simulink library "tqd"  (R2021b)
settings: Solver=VariableStepAuto  StartTime=0.0  StopTime=10.0  RelTol=1e-3
undefined symbols (not defined in the file): ATQD_AfterTqMinGain_X_Deg, ATQD_APSCreepBaseTqD_X_kph, ATQD_APSCreepBaseTqD_Y_Deg, ATQD_APSCreepBaseTqR_X_kph, ATQD_APSCreepBaseTqR_Y_Deg, ATQD_APSCreepIterm_X_kph, ATQD_APSCreepIterm_Y_kph, ATQD_APSCreepPterm_X_kph, ATQD_APSCreepPterm_Y_kph, ATQD_APSDecReq_X_kph, ATQD_APSDecReq_Y_mps2, ATQD_APSDecReqCMD_X_kph, ATQD_APSDecReqTs_X_pct, ATQD_APSDecTimeGain_X_Deg, ATQD_APSDecTimeGain_Y_s, ATQD_APSReqLowSpd_X_Deg, ATQD_AutoHoldReleaseBPS_X_Deg, ATQD_AWDLoadTrqnsGain_X_kg, ATQD_AWDLoadTrqnsGain_Y_pct, ATQD_BOSEnBPSPosn_X_kph, ATQD_BOSMap_X_rpm, ATQD_BOSMap_Y_pct, ATQD_CreepBaseTqD_X_kph, ATQD_CreepBaseTqD_Y_Deg, ATQD_CreepBaseTqR_X_kph, ATQD_CreepBaseTqR_Y_Deg, ATQD_CreepBPSDisPosn_X_Deg, ATQD_CreepBPSDisPosnR_X_Deg, ATQD_CreepBPSEnPosn_X_Deg, ATQD_CreepBPSEnPosnR_X_Deg, ATQD_CreepDeltaTq_X_kph, ATQD_CreepIterm_X_kph, ATQD_CreepIterm_Y_kph, ATQD_CreepItermMaxLimit_X_pct, ATQD_CreepPreloadTime_X_kph, ATQD_CreepPreloadTq_X_kph, ATQD_CreepPreloadTq_Y_s, ATQD_CreepProtTq_X_Deg, ATQD_CreepPterm_X_kph, ATQD_CreepPterm_Y_kph, ATQD_CreepRrTqSpRat_X_rpm, ATQD_CreepRrTqSpRat_Y_Nm, ATQD_CreepTargetSpdD_X_pct, ATQD_CreepTargetSpdR_X_pct, ATQD_ECOTqMapD_X_rpm, ATQD_ECOTqMapD_Y_pct, ATQD_EMTqMapD_X_rpm, ATQD_EMTqMapD_Y_pct, ATQD_EOPDTqMapDCon_X_rpm, ATQD_EOPDTqMapDCon_Y_Deg, ATQD_EscapeModePedTq_X_pct, ATQD_EscapeModePedTq_Y_rpm, ATQD_EscapeModePedTqFr_X_pct, ATQD_EscapeModePedTqFr_Y_rpm, ATQD_EstInitVehWeight_X_c, ATQD_FAfterTqCMDGain_X_rpm, ATQD_FAfterTqCMDGain_Y_pct, ATQD_FrLossMAPLowV_X_rpm, ATQD_FrLossMAPLowV_Y_Nm, ATQD_FrMotActReduce_X_rpm ... (+772)
libraries: simulink x211, hcu_lib x179, tqr x3
(part 7 of 28)

== system tqd/TQD/TorqueDemand/Signal_convert/SWC2_Subsystem ==
  note: Speed Setting Mode
  note: Speed Control Mode
  note: Fail safe switch
  VINP_SWC2LScrollUpSta_flg : Inport
  VINP_SWC2LScrollDownSta_flg : Inport  Port=2
  VINP_SWC2LScrollPressSta_flg : Inport  Port=3
  VINP_SWC2LADASSta_flg : Inport  Port=4
  VTQD_GearActualPosn_enum : Inport  Port=5
  VVMC_ADASActive_flg : Inport  Port=6
  VVMC_LVDAACCStaInfor_flg : Inport  Port=7
  VVMC_MSAActive_flg : Inport  Port=8
  VINP_ADASACCSta_enum : Inport  Port=9
  VVMC_MeterIndSpeed_raw32 : Inport  Port=10
  VINP_ADASSLIFSpdLim_enum : Inport  Port=11
  task_time_s : Inport  Port=12
  VINP_IVIISAOffsetSpd_enum : Inport  Port=13
  VPMM_PowerSta_enum : Inport  Port=14
  VTQD_ShiftGearPosn_enum : Inport  Port=15
  VVMC_MSACtrlSta_enum : Inport  Port=16
  VINP_VehSpeed_kph : Inport  Port=17
  VINP_Distanceunit_flg : Inport  Port=18
  VINP_IVIACCAdaptiveSta_flg : Inport  Port=19
  VVMC_CCCtrlSta_enum : Inport  Port=20
  VVMC_ACCObjDist_m : Inport  Port=21
  VINP_SmartEcoModeSW_flg : Inport  Port=22
  VVMC_SetACCDisableAPS_flg : Inport  Port=23
  VINP_SWCRegenUp_flg : Inport  Port=24
  VINP_SWCRegenDown_flg : Inport  Port=25
  VINP_SWC2RScrollUpSta_flg : Inport  Port=26
  VINP_SWC2RScrollDownSta_flg : Inport  Port=27
  VINP_SWC2LDriveModeSta_flg : Inport  Port=28
  VINP_SWC2RScrollPressSta_flg : Inport  Port=29
  VINP_SWC2RRightSta_flg : Inport  Port=30
  VINP_SWC2RLeftSta_flg : Inport  Port=31
  VTQD_LowIdleAccPedal_flg : Inport  Port=32
  Enable : EnablePort
  AND1 : Logic  AllPortsSameDT=off  OutDataTypeStr=boolean
  AND{8,10,12..13,17..18} (6 alike) : Logic  Inputs=3  AllPortsSameDT=off  OutDataTypeStr=boolean
  AND11 : Logic  Inputs=4  AllPortsSameDT=off  OutDataTypeStr=boolean
  AND14 : Logic  Operator=OR  AllPortsSameDT=off  OutDataTypeStr=boolean
  AND16 : Logic  Operator=OR  AllPortsSameDT=off  OutDataTypeStr=boolean
  AND6 : Logic  AllPortsSameDT=off  OutDataTypeStr=boolean
  Add1 : Sum
  Big Mike Combo : Subsystem  AncestorBlock=tqd0/TQD/TorqueDemand/Signal_convert/Big Mike Combo
  Constant1 : Constant  Value=ENUM_ADASACCSTA_OVERRIDE
  Constant{89,92,94..95,110..113} (8 alike) : Constant  Value=FALSE
  Constant116 : Constant  Value=ENUM_GEARACTUALPOSN_D
  Constant117 : Constant  Value=ENUM_SWCBOTTONPRESS_LONGPRESS
  Constant118 : Constant  Value=ENUM_GEARACTUALPOSN_D
  Constant119 : Constant  Value=ENUM_SPDCTRLMODE_MSA
  Constant120 : Constant  Value=ENUM_SWCBOTTONPRESS_SHORTPRESS
  Constant121 : Constant  Value=KTQD_OvrSpdSetDownOffSet_kph
  Constant122 : Constant  Value=ENUM_SWCBOTTONPRESS_LONGPRESS
  Constant123 : Constant  Value=ENUM_SWCBOTTONPRESS_SHORTPRESS
  Constant124 : Constant  Value=ENUM_ADASACCSTA_ACTIVE
  Constant125 : Constant  Value=ENUM_ADASACCSTA_ACTIVE
  Constant126 : Constant  Value=0x0  OutDataTypeStr=uint8
  Constant127 : Constant  Value=ENUM_SPDCTRLMODE_MSA
  Constant128 : Constant  Value=ENUM_SPDCTRLMODE_ACC
  Constant129 : Constant  Value=ENUM_GEARACTUALPOSN_D
  Constant130 : Constant  Value=ENUM_SPDCTRLMODE_MSA
  Constant77 : Constant  Value=KTQD_SpdCtrlMode_enum_ovrdflg
  Constant78 : Constant  Value=KTQD_SpdCtrlMode_enum_ovrdval
  Constant82 : Constant  Value=KTQD_Veh2MetSpdLowBand_kph
  Constant84 : Constant  Value=KTQD_Veh2MetSpdHiBand_kph
  Constant90 : Constant  Value=ENUM_POWERSTA_READY
  Constant91 : Constant  Value=ENUM_SPDCTRLMODE_OFF
  Data Type Conversion4 : DataTypeConversion  OutDataTypeStr=single
  Delay{5..6,10..13} (6 alike) : Delay  DelayLength=1
  Detect Decrease2 : simulink/Logic and Bit Operations/Detect Decrease  vinit=0.0  OutDataTypeStr=boolean
  Detect Increase1 : simulink/Logic and Bit Operations/Detect Increase  vinit=0.0  OutDataTypeStr=boolean
  Detect Increase2 : simulink/Logic and Bit Operations/Detect Increase  vinit=0.0  OutDataTypeStr=boolean
  Equal{1,30,41..48,50,52} (12 alike) : RelationalOperator  Operator===  OutDataTypeStr=boolean  RndMeth=Simplest
  Equal{40,49,51,53} (4 alike) : RelationalOperator  Operator=~=  OutDataTypeStr=boolean  RndMeth=Simplest
  L_ScrollPress Behavior : Subsystem
  NOT{1..4} (4 alike) : Logic  Operator=NOT  AllPortsSameDT=off  OutDataTypeStr=boolean
  OR2 : Logic  Operator=OR  Inputs=4  AllPortsSameDT=off  OutDataTypeStr=boolean
  OR{3..8} (6 alike) : Logic  Operator=OR  AllPortsSameDT=off  OutDataTypeStr=boolean
  Relational Operator2 : RelationalOperator  OutDataTypeStr=boolean  RndMeth=Simplest
  Relational Operator3 : RelationalOperator  Operator=>  OutDataTypeStr=boolean  RndMeth=Simplest
  Relational Operator6 : RelationalOperator  Operator=<=  OutDataTypeStr=boolean  RndMeth=Simplest
  Road Speed Limit Convert : Subsystem
  SR_Latch4 : hcu_lib/Basic_Blocks/SR_Latch
  SR_Latch9 : hcu_lib/Basic_Blocks/SR_Latch
  Speed Control Mode : Stateflow chart  AncestorBlock=tqd0/TQD/TorqueDemand/Signal_convert/Speed Control Mode  TreatAsAtomicUnit=on
  Speed Setting Mode : Subsystem
  Switch{13,15..16,23..26} (7 alike) : Switch  Criteria=u2 ~= 0
  Switch19 : Switch  Criteria=u2 > Threshold
  Terminator{,1..5} (6 alike) : Terminator
  VTQD_IVIISAOffsetSpdCHOOSE_flg : Subsystem
  Vehicle to Meter Speed : Subsystem
  VTQD_SWC2ResUpSta_flg : Outport
  VTQD_SWC2SetdownSta_flg : Outport  Port=2
  VTQD_SWC2CancelSta_flg : Outport  Port=3
  VTQD_SWC2LADASSta_flg : Outport  Port=4
  VTQD_SpdLim4SetSpd_raw32 : Outport  Port=5
  VTQD_SWC2SetSpdLimWarn_flg : Outport  Port=6
  VTQD_SpdCtrlMode_enum : Outport  Port=7
  VTQD_SpdCtrlSta_flg : Outport  Port=8
  VTQD_SetSpd_kph : Outport  Port=9
  VTQD_SWC2ACCSetSpd_kph : Outport  Port=10
  VTQD_SWC2CCSetSpd_kph : Outport  Port=11
  VTQD_SWC2MSASetSpd_kph : Outport  Port=12
  VTQD_SWC2ISASetSpd_kph : Outport  Port=13
  VTQD_SWC2AllowSetSpd_flg : Outport  Port=14
  VTQD_SWC2CCSpdResetFinish_flg : Outport  Port=15
  VTQD_ComboKeyPreEn_flg : Outport  Port=16
  VTQD_ComboKeyEn_flg : Outport  Port=17
  VTQD_SysMode_enum : Outport  Port=18
  wires:
  Detect Increase2/1 -> OR6/2
  [VTQD_SWC2SetDownSta_flg] -> Speed Setting Mode/16(VTQD_SWC2SetDownSta_flg)
  Constant130/1 -> Equal52/2
  Switch19/1 -> VTQD_SpdLim4SetSpd_raw32/1, [VTQD_SpdLim4SetSpd_raw32]  "VTQD_SpdLim4SetSpd_raw32"
  Switch23/1 -> [VTQD_SWC2ScrollUpSta_flg]  "VTQD_SWC2ScrollUpSta_flg"
  [VINP_IVIISAOffsetSpd_enum] -> Road Speed Limit Convert/2(VINP_IVIISAOffsetSpd_enum)
  [VPMM_PowerSta_enum] -> Speed Setting Mode/1(VPMM_PowerSta_enum)
  Switch13/1 -> Switch15/1
  Switch24/1 -> Terminator/1
  [VDDM_SWC2LADASSta_flg] -> Switch16/2
  AND11/1 -> OR2/1
  Delay11/1 -> Equal45/1
  [VINP_ADASSLIFSpdLim_enum] -> Equal53/1
  SR_Latch4/1 -> OR3/2
  [VTQD_SWC2LADASSta_flg] -> Detect Increase2/1
  [VVMC_MeterIndSpeed_raw32] -> Speed Setting Mode/23(VVMC_MeterIndSpeed_raw32)
  NOT2/1 -> SR_Latch9/2
  Switch16/1 -> VTQD_SWC2LADASSta_flg/1, [VTQD_SWC2LADASSta_flg]  "VTQD_SWC2LADASSta_flg"
  [VTQD_LScrollPressShort_flg] -> AND17/2
  Constant118/1 -> Equal42/2
  Equal48/1 -> OR4/2
  [VVMC_MeterIndSpeed_raw32] -> Switch19/3
  [VTQD_SWC2LScrollPressSta_flg] -> NOT2/1
  [VTQD_IVIISAOffsetSpdCHOOSE_flg] -> Road Speed Limit Convert/3(VTQD_IVIISAOffsetSpdCHOOSE_flg)
  AND18/1 -> OR3/1
  [VVMC_LVDAACCStaInfor_flg] -> AND8/2
  Delay13/1 -> Equal49/1
  [VTQD_LScrollPressLong_flg] -> Speed Control Mode/2(VTQD_LScrollPressLong_flg)
  [VTQD_RoadSpdLim_raw32] -> Switch19/1
  [VINP_ADASACCSta_enum] -> Speed Setting Mode/4(VINP_ADASACCSta_enum)
  [VINP_IVIACCAdaptiveSta_flg] -> Speed Setting Mode/19(VINP_IVIACCAdaptiveSta_flg)
  [VINP_SmartEcoModeSW_flg] -> Speed Setting Mode/17(VINP_SmartEcoModeSW_flg)
  [VINP_Distanceunit_flg] -> Speed Setting Mode/14(VINP_Distanceunit_flg)
  [VINP_IVIACCAdaptiveSta_flg] -> OR7/1
  [VVMC_SetACCDisableAPS_flg] -> Speed Setting Mode/18(VVMC_SetACCDisableAPS_flg)
  Speed Setting Mode/3(VTQD_SWC2SetSpdLimWarn_flg) -> VTQD_SWC2SetSpdLimWarn_flg/1
  [VVMC_LVDAACCStaInfor_flg] -> Speed Setting Mode/11(VVMC_LVDAACCStatusInformation_flg)
  [VTQD_SWC2ScrollDownSta_flg] -> Speed Setting Mode/9(VTQD_SWC2ScrollDownSta_flg)
  Switch15/1 -> VTQD_SpdCtrlMode_enum/1, [VTQD_SpdCtrlMode_enum]
  [task_time_s] -> Speed Setting Mode/10(task_time_s)
  [VTQD_SWC2ScrollUpSta_flg] -> Speed Setting Mode/8(VTQD_SWC2ScrollUpSta_flg)
  [VVMC_ACCObjDist_m] -> Speed Setting Mode/12(VVMC_ACCObjDist_m)
  OR4/1 -> AND13/3
  Relational Operator2/1 -> AND6/1
  OR7/1 -> Switch19/2
  Detect Increase1/1 -> OR6/1
  [task_time_s] -> L_ScrollPress Behavior/2(TASK_TIME)
  Equal43/1 -> AND11/3
  [VTQD_SetRoadSpdLim_flg] -> Speed Setting Mode/21(VTQD_SetRoadSpdLim_flg)
  [VTQD_SpdCtrlMode_enum] -> Speed Setting Mode/3(VTQD_SpdCtrlMode_enum)
  [VVMC_MSACtrlSta_enum] -> Speed Setting Mode/6(VVMC_MSACtrlSta_enum)
  [VTQD_SpdCtrlMode_enum] -> Equal44/1
  [VTQD_SetRoadSpdLim_flg] -> OR7/2
  Speed Control Mode/2(VTQD_SpdCtrlSta_flg) -> VTQD_SpdCtrlSta_flg/1
  Equal50/1 -> AND10/2
  [VVMC_CCCtrlSta_enum] -> Speed Setting Mode/5(VVMC_CCCtrlSta_enum)
  [VTQD_ShiftGearPosn_enum] -> Speed Control Mode/3(VTQD_ShiftGearPosn_enum)
  Relational Operator3/1 -> AND13/1
  [VVMC_MSACtrlSta_enum] -> Speed Control Mode/5(VVMC_MSACtrlSta_enum)
  [VTQD_ShiftGearPosn_enum] -> Road Speed Limit Convert/5(VTQD_ShiftGearPosn_enum)
  NOT4/1 -> AND11/4
  Delay12/1 -> Equal40/1
  [VINP_Distanceunit_flg] -> Road Speed Limit Convert/4(VINP_Distanceunit_flg)
  [VTQD_SWC2LADASSta_flg] -> Speed Control Mode/4(VTQD_SWC2LADASSta_flg)
  Constant82/1 -> Relational Operator2/2
  [VINP_ADASSLIFSpdLim_enum] -> Road Speed Limit Convert/1(VINP_ADASSLIFSpdLim_enum)
  AND10/1 -> OR2/2
  NOT1/1 -> AND11/1
  [VTQD_SpdLim4SetSpd_raw32] -> Speed Setting Mode/13(VTQD_SpdLim4SetSpd_raw32)
  Constant129/1 -> Equal51/2
  [VPMM_PowerSta_enum] -> Speed Control Mode/1(VPMM_PowerSta_enum)
  Constant121/1 -> Add1/1
  [VTQD_LScrollPressLong_flg] -> AND12/1
  [VVMC_ADASActive_flg] -> AND16/1
  Equal49/1 -> AND10/1
  Speed Setting Mode/2(VTQD_SWC2ScrollUpSta_enum) -> [VTQD_SWC2ScrollUpSta_enum]
  Constant92/1 -> Switch25/1
  AND12/1 -> SR_Latch9/1
  [VTQD_GearActualPosn_enum] -> Equal51/1
  [VVMC_MSAActive_flg] -> AND16/2
  OR5/1 -> VTQD_SWC2CancelSta_flg/1, [VTQD_SWC2CANCELSta_flg]  "VTQD_SWC2CancelSta_flg"
  Equal47/1 -> OR4/1
  Constant126/1 -> Equal53/2
  Equal53/1 -> AND17/3
  [VTQD_SetSpd_kph] -> Delay5/1
  [VTQD_LScrollPressLong_flg] -> AND11/2
  Constant120/1 -> Equal45/2
  Constant125/1 -> Equal50/2
  Constant123/1 -> Equal48/2
  [VVMC_MeterIndSpeed_raw32] -> Relational Operator3/1
  L_ScrollPress Behavior/2("VTQD_LScrollPressLong_flg\t") -> [VTQD_LScrollPressLong_flg]  "VTQD_LScrollPressLong_flg"
  Constant117/1 -> Equal41/2
  Constant124/1 -> Equal49/2
  [VTQD_SWC2ScrollUpSta_enum] -> Delay11/1
  OR8/1 -> Detect Decrease2/1
  Constant127/1 -> Equal43/2
  [VTQD_SWC2CANCELSta_flg] -> NOT1/1
  [VINP_ADASACCSta_enum] -> Delay13/1
  Delay5/1 -> Add1/2
  [VVMC_ADASActive_flg] -> AND8/1
  Equal46/1 -> AND10/3
  Detect Decrease2/1 -> SR_Latch4/2
  Constant116/1 -> Equal40/2
  Add1/1 -> Relational Operator3/2
  Equal40/1 -> AND18/1
  [VTQD_GearActualPosn_enum] -> Equal42/1
  AND13/1 -> OR2/3, [VTQD_Set2MeterSpd_flg]  "VTQD_Set2MeterSpd_flg"
  AND14/1 -> AND13/2
  [VDDM_SWC2LScrollPressSta_flg] -> Switch26/2
  [VINP_SWC2LADASSta_flg] -> Switch16/3
  Equal30/1 -> Switch15/2
  Equal44/1 -> AND18/3
  [VINP_SWC2LScrollPressSta_flg] -> Switch26/3
  [VINP_ADASSLIFSpdLim_enum] -> Speed Setting Mode/7(VINP_ADASSLIFSpdLim_enum)
  Equal45/1 -> OR8/2
  [VTQD_Set2MeterSpd_flg] -> Speed Setting Mode/20(VTQD_Set2MeterSpd_flg)
  Constant94/1 -> Switch26/1
  Constant90/1 -> Equal30/2
  Data Type Conversion4/1 -> VTQD_SetSpd_kph/1, [VTQD_SetSpd_kph]
  [VINP_IVIISAOffsetSpd_enum] -> VTQD_IVIISAOffsetSpdCHOOSE_flg/1(VTQD_IVIISAOffsetSpd_enum)
  [VINP_VehSpeed_kph] -> Relational Operator6/1
  Constant77/1 -> Switch13/2
  Speed Control Mode/1(VTQD_SpdCtrlMode_enum) -> Switch13/3
  [VINP_VehSpeed_kph] -> Relational Operator2/1
  [VTQD_SpdCtrlMode_enum] -> Equal46/1
  L_ScrollPress Behavior/1(VTQD_LScrollPressShort_flg) -> [VTQD_LScrollPressShort_flg]  "VTQD_LScrollPressShort_flg"
  [VPMM_PowerSta_enum] -> Equal30/1
  VTQD_IVIISAOffsetSpdCHOOSE_flg/1(VTQD_IVIISAOffsetSpdCHOOSE_flg) -> [VTQD_IVIISAOffsetSpdCHOOSE_flg]
  [VTQD_SWC2LScrollPressSta_flg] -> L_ScrollPress Behavior/1(VTQD_SWC2LScrollPressSta_flg)
  [VVMC_MSAActive_flg] -> AND12/2
  Equal41/1 -> OR8/1
  Constant119/1 -> Equal44/2
  Constant122/1 -> Equal47/2
  [VINP_SWC2LScrollDownSta_flg] -> Switch25/3
  Equal42/1 -> AND18/2
  Relational Operator6/1 -> AND6/2
  Road Speed Limit Convert/1(VTQD_RoadSpdLim_raw32) -> [VTQD_RoadSpdLim_raw32]
  SR_Latch9/1 -> OR5/2
  [VVMC_MSAActive_flg] -> NOT4/1
  Delay10/1 -> Equal41/1
  [VTQD_SWC2ScrollUpSta_enum] -> Equal47/1
  AND8/1 -> SR_Latch4/1
  [VTQD_SpdCtrlMode_enum] -> Equal52/1
  AND6/1 -> Switch24/2
  [VTQD_SWC2ScrollUpSta_enum] -> Equal48/1
  [VINP_SWC2LScrollUpSta_flg] -> Switch23/3
  Constant95/1 -> Switch16/1
  Equal52/1 -> AND12/3
  Equal51/1 -> OR5/1
  OR6/1 -> AND8/3
  [VTQD_SWC2ScrollUpSta_flg] -> Detect Increase1/1
  Constant128/1 -> Equal46/2
  [VDDM_SWC2LScrollUpSta_flg] -> Switch23/2
  [VINP_VehSpeed_kph] -> Switch24/3
  Vehicle to Meter Speed/1(OutputSpeed) -> Switch24/1
  [VTQD_SpdCtrlMode_enum] -> Equal43/1
  Constant78/1 -> Switch13/1
  AND17/1 -> [VTQD_SetRoadSpdLim_flg], OR2/4  "VTQD_SetRoadSpdLim_flg"
  Constant84/1 -> Relational Operator6/2
  [VTQD_ShiftGearPosn_enum] -> Speed Setting Mode/2(VTQD_ShiftGearPosn_enum)
  [VDDM_SWC2LScrollDownSta_flg] -> Switch25/2
  [VTQD_SWC2ResUpSta_flg] -> Speed Setting Mode/15(VTQD_SWC2ResUpSta_flg)
  [VINP_VehSpeed_kph] -> Vehicle to Meter Speed/1(InputSpeed)
  Constant89/1 -> Switch23/1
  [VINP_ADASACCSta_enum] -> Equal50/1
  Constant91/1 -> Switch15/3
  Switch26/1 -> [VTQD_SWC2LScrollPressSta_flg]  "VTQD_SWC2LScrollPressSta_flg"
  OR3/1 -> VTQD_SWC2ResUpSta_flg/1, [VTQD_SWC2ResUpSta_flg]  "VTQD_SWC2ResUpSta_flg"
  Switch25/1 -> [VTQD_SWC2ScrollDownSta_flg]  "VTQD_SWC2ScrollDownSta_flg"
  [VTQD_GearActualPosn_enum] -> Delay12/1
  Speed Setting Mode/1(VTQD_SetSpd_kph) -> Data Type Conversion4/1
  [VTQD_SWC2ScrollUpSta_enum] -> Delay10/1
  [VTQD_LScrollPressShort_flg] -> Speed Setting Mode/22(VTQD_LScrollPressShort_flg)
  OR2/1 -> VTQD_SWC2SetdownSta_flg/1, [VTQD_SWC2SetDownSta_flg]  "VTQD_SWC2SetdownSta_flg"
  AND16/1 -> AND17/1
  VINP_ADASACCSta_enum/1 -> [VINP_ADASACCSta_enum]
  VTQD_GearActualPosn_enum/1 -> [VTQD_GearActualPosn_enum]
  VINP_ADASSLIFSpdLim_enum/1 -> [VINP_ADASSLIFSpdLim_enum]
  task_time_s/1 -> [task_time_s]
  VVMC_MSACtrlSta_enum/1 -> [VVMC_MSACtrlSta_enum]
  VINP_SWC2LADASSta_flg/1 -> [VINP_SWC2LADASSta_flg]
  VVMC_SetACCDisableAPS_flg/1 -> [VVMC_SetACCDisableAPS_flg]
  VINP_VehSpeed_kph/1 -> [VINP_VehSpeed_kph]
  VPMM_PowerSta_enum/1 -> [VPMM_PowerSta_enum]
  VINP_SmartEcoModeSW_flg/1 -> [VINP_SmartEcoModeSW_flg]
  VINP_IVIACCAdaptiveSta_flg/1 -> [VINP_IVIACCAdaptiveSta_flg]
  VVMC_CCCtrlSta_enum/1 -> [VVMC_CCCtrlSta_enum]
  VINP_Distanceunit_flg/1 -> [VINP_Distanceunit_flg]
  VINP_SWC2LScrollUpSta_flg/1 -> [VINP_SWC2LScrollUpSta_flg]
  VVMC_LVDAACCStaInfor_flg/1 -> [VVMC_LVDAACCStaInfor_flg]
  VVMC_MeterIndSpeed_raw32/1 -> [VVMC_MeterIndSpeed_raw32]
  VVMC_MSAActive_flg/1 -> [VVMC_MSAActive_flg]
  VVMC_ACCObjDist_m/1 -> [VVMC_ACCObjDist_m]
  VVMC_ADASActive_flg/1 -> [VVMC_ADASActive_flg]
  VINP_IVIISAOffsetSpd_enum/1 -> [VINP_IVIISAOffsetSpd_enum]
  VINP_SWC2LScrollPressSta_flg/1 -> [VINP_SWC2LScrollPressSta_flg]
  VTQD_ShiftGearPosn_enum/1 -> [VTQD_ShiftGearPosn_enum]
  VINP_SWC2LScrollDownSta_flg/1 -> [VINP_SWC2LScrollDownSta_flg]
  Speed Setting Mode/4(VTQD_SWC2ACCSetSpd_kph) -> VTQD_SWC2ACCSetSpd_kph/1
  Speed Setting Mode/5(VTQD_SWC2CCSetSpd_kph) -> VTQD_SWC2CCSetSpd_kph/1
  Speed Setting Mode/6(VTQD_SWC2MSASetSpd_kph) -> VTQD_SWC2MSASetSpd_kph/1
  Speed Setting Mode/7(VTQD_SWC2ISASetSpd_kph) -> VTQD_SWC2ISASetSpd_kph/1
  Speed Setting Mode/8(VTQD_SWC2AllowSetSpd_flg) -> VTQD_SWC2AllowSetSpd_flg/1
  Speed Setting Mode/9(VTQD_SWC2CCSpdResetFinish_flg) -> VTQD_SWC2CCSpdResetFinish_flg/1
  Constant113/1 -> [VDDM_SWC2LADASSta_flg]  "VDDM_SWC2LADASSta_flg"
  Constant111/1 -> [VDDM_SWC2LScrollDownSta_flg]  "VDDM_SWC2LScrollDownSta_flg"
  Constant110/1 -> [VDDM_SWC2LScrollUpSta_flg]  "VDDM_SWC2LScrollUpSta_flg"
  Constant112/1 -> [VDDM_SWC2LScrollPressSta_flg]  "VDDM_SWC2LScrollPressSta_flg"
  [VINP_SWC2LScrollUpSta_flg] -> Big Mike Combo/4(VINP_SWC2LScrollUpSta_flg)
  Big Mike Combo/1(VTQD_StreetFightMode_flg) -> Terminator1/1
  [VPMM_PowerSta_enum] -> Big Mike Combo/14(VPMM_PowerSta_enum)
  Big Mike Combo/5(VTQD_ManufactureMode_flg) -> Terminator3/1
  Delay6/1 -> Big Mike Combo/15(VTQD_ShiftGearPosn_enum)  "VTQD_ShiftGearPosn_enum"
  Big Mike Combo/4(VTQD_EngineeringMode_flg) -> Terminator2/1
  Big Mike Combo/6(VTQD_ExhibitionMode_flg) -> Terminator4/1
  [VINP_SWC2LScrollPressSta_flg] -> Big Mike Combo/8(VINP_SWC2LScrollPressSta_flg)
  [VTQD_ShiftGearPosn_enum] -> Delay6/1
  [VINP_SWC2LScrollDownSta_flg] -> Big Mike Combo/5(VINP_SWC2LScrollDownSta_flg)
  Big Mike Combo/2(VTQD_ComboKeyPreEn_flg) -> VTQD_ComboKeyPreEn_flg/1
  [task_time_s] -> Big Mike Combo/1(task_time_s)
  Big Mike Combo/8(VTQD_SysMode_enum) -> VTQD_SysMode_enum/1
  [VINP_SWC2LADASSta_flg] -> Big Mike Combo/9(VINP_SWC2LADASSta_flg)
  Big Mike Combo/7(VTQD_DiagnosisOffMode_flg) -> Terminator5/1  "VSCP_DiagnosisOffMode_flg"
  Big Mike Combo/3(VTQD_ComboKeyEn_flg) -> VTQD_ComboKeyEn_flg/1
  VINP_SWC2RScrollDownSta_flg/1 -> [VINP_SWC2RScrollDownSta_flg]
  VINP_SWCRegenUp_flg/1 -> [VINP_SWCRegenUp_flg]
  VINP_SWC2RScrollUpSta_flg/1 -> [VINP_SWC2RScrollUpSta_flg]
  VINP_SWCRegenDown_flg/1 -> [VINP_SWCRegenDown_flg]
  VINP_SWC2LDriveModeSta_flg/1 -> [VINP_SWC2LDriveModeSta_flg]
  VINP_SWC2RScrollPressSta_flg/1 -> [VINP_SWC2RScrollPressSta_flg]
  VINP_SWC2RLeftSta_flg/1 -> [VINP_SWC2RLeftSta_flg]
  VINP_SWC2RRightSta_flg/1 -> [VINP_SWC2RRightSta_flg]
  [VINP_SWCRegenUp_flg] -> Big Mike Combo/2(VINP_SWC2RegenDown_flg)
  [VINP_SWCRegenDown_flg] -> Big Mike Combo/3(VINP_SWC2RegenUp_flg)
  [VINP_SWC2RLeftSta_flg] -> Big Mike Combo/13(VINP_SWC2RLeftSta_flg)
  [VINP_SWC2RRightSta_flg] -> Big Mike Combo/12(VINP_SWCRightSta_flg)
  [VINP_SWC2RScrollPressSta_flg] -> Big Mike Combo/11(VINP_SWC2RScrollPressSta_flg)
  [VINP_SWC2LDriveModeSta_flg] -> Big Mike Combo/10(VINP_SWC2LDriveModeSta_flg)
  [VINP_SWC2RScrollDownSta_flg] -> Big Mike Combo/7(VINP_SWCDownSta_flg)
  [VINP_SWC2RScrollUpSta_flg] -> Big Mike Combo/6(VINP_SWC2RScrollUpSta_flg)
  NOT3/1 -> AND1/2
  Constant1/1 -> Equal1/2
  [VINP_ADASACCSta_enum] -> Equal1/1
  [VVMC_MSAActive_flg] -> AND1/1
  [VTQD_LowIdleAccPedal_flg] -> NOT3/1
  Equal1/1 -> AND14/1
  AND1/1 -> AND14/2
  VTQD_LowIdleAccPedal_flg/1 -> [VTQD_LowIdleAccPedal_flg]
  [VVMC_MSACtrlSta_enum] -> L_ScrollPress Behavior/3(VVMC_MSACtrlSta_enum)

== system tqd/TQD/TorqueDemand/Signal_convert/SWC_Subsystem ==
  note: Speed Control Mode
  note: Speed Setting Mode
  VDDM_SWCResUpSta_flg : Inport
  VINP_SWCResUpSta_flg : Inport  Port=2
  VDDM_SWCSetdownSta_flg : Inport  Port=3
  VINP_SWCSetdownSta_flg : Inport  Port=4
  VDDM_SWCACCSta_flg : Inport  Port=5
  VINP_SWCACCSta_flg : Inport  Port=6
  VDDM_SWCCANCELSta_flg : Inport  Port=7
  VINP_SWCCANCELSta_flg : Inport  Port=8
  VTQD_IVIISAOffsetSpd_enum : Inport  Port=9
  VPMM_PowerSta_enum : Inport  Port=10
  VINP_ADASACCSta_enum : Inport  Port=11
  VINP_ADASISASta_enum : Inport  Port=12
  VTQD_ShiftGearPosn_enum : Inport  Port=13
  VINP_VehSpeed_kph : Inport  Port=14
  VVMC_CCCtrlSta_enum : Inport  Port=15
  VVMC_MSACtrlSta_enum : Inport  Port=16
  VINP_ADASVehSpdLim_kph : Inport  Port=17
  task_time_s : Inport  Port=18
  VVMC_LVDAACCStatusInformation_flg : Inport  Port=19
  VVMC_ACCObjDist_m : Inport  Port=20
  VVMC_MeterIndSpeed_raw32 : Inport  Port=21
  VINP_Distanceunit_flg : Inport  Port=22
  VINP_SmartEcoModeSW_flg : Inport  Port=23
  VVMC_SetACCDisableAPS_flg : Inport  Port=24
  Enable : EnablePort
  AND6 : Logic  AllPortsSameDT=off  OutDataTypeStr=boolean
  Constant77 : Constant  Value=KTQD_SpdCtrlMode_enum_ovrdflg
  Constant78 : Constant  Value=KTQD_SpdCtrlMode_enum_ovrdval
  Constant82 : Constant  Value=KTQD_Veh2MetSpdLowBand_kph
  Constant84 : Constant  Value=KTQD_Veh2MetSpdHiBand_kph
  Constant{89,92,94..95} (4 alike) : Constant  Value=FALSE
  Constant90 : Constant  Value=ENUM_POWERSTA_READY
  Constant91 : Constant  Value=ENUM_SPDCTRLMODE_OFF
  Data Type Conversion4 : DataTypeConversion  OutDataTypeStr=single
  Equal30 : RelationalOperator  Operator===  OutDataTypeStr=boolean  RndMeth=Simplest
  Relational Operator2 : RelationalOperator  OutDataTypeStr=boolean  RndMeth=Simplest
  Relational Operator6 : RelationalOperator  Operator=<=  OutDataTypeStr=boolean  RndMeth=Simplest
  SpdCtrlBotton Behavior : Subsystem
  Speed Control Mode : Stateflow chart  TreatAsAtomicUnit=on
  Speed Setting Mode : Subsystem
  Switch{13,15..16,23..26} (7 alike) : Switch  Criteria=u2 ~= 0
  Terminator : Terminator
  VTQD_IVIISAOffsetSpdCHOOSE_flg : Subsystem
  Vehicle to Meter Speed : Subsystem
  VTQD_SWCResUpSta_flg : Outport
  VTQD_SWCSetdownSta_flg : Outport  Port=2
  VTQD_SWCCancelSta_flg : Outport  Port=3
  VTQD_SWCSetSpdLimWarn_flg : Outport  Port=4
  VTQD_SWCSpdCtrlMode_enum : Outport  Port=5
  VTQD_SWCSpdCtrlSta_flg : Outport  Port=6
  VTQD_SWCSetSpd_kph : Outport  Port=7
  VTQD_SWCACCSetSpd_kph : Outport  Port=8
  VTQD_SWCCCSetSpd_kph : Outport  Port=9
  VTQD_SWCMSASetSpd_kph : Outport  Port=10
  VTQD_SWCISASetSpd_kph : Outport  Port=11
  VTQD_SWCAllowSetSpd_flg : Outport  Port=12
  VTQD_SWCCCSpdResetFinish_flg : Outport  Port=13
  wires:
  VDDM_SWCACCSta_flg/1 -> Switch26/2
  [VTQD_SpdCtrlMode_enum] -> Speed Setting Mode/3(VTQD_SpdCtrlMode_enum)
  VVMC_ACCObjDist_m/1 -> Speed Setting Mode/13(VVMC_ACCObjDist_m)
  VINP_ADASVehSpdLim_kph/1 -> Speed Setting Mode/7(VINP_ADASVehSpdLim_kph)
  Constant77/1 -> Switch13/2
  VINP_SWCResUpSta_flg/1 -> Switch23/3
  Speed Setting Mode/1(VTQD_SetSpd_kph) -> Data Type Conversion4/1
  Constant89/1 -> Switch23/1
  [task_time_s] -> SpdCtrlBotton Behavior/2(TASK_TIME)
  SpdCtrlBotton Behavior/2("VTQD_SpdCtrlLongP_flg\t") -> [VTQD_SpdCtrlLongP_flg]  "VTQD_SpdCtrlLongP_flg"
  VINP_ADASISASta_enum/1 -> Speed Control Mode/5(VINP_ADASISASta_enum)
  Constant92/1 -> Switch25/1
  [VTQD_SWCResUpSta_flg] -> Speed Setting Mode/8(VTQD_SWCResUpSta_flg)
  Switch26/1 -> [VTQD_SWCACCSta_flg]  "VTQD_SWCACCSta_flg"
  Constant91/1 -> Switch15/3
  VDDM_SWCResUpSta_flg/1 -> Switch23/2
  VINP_SWCACCSta_flg/1 -> Switch26/3
  Constant95/1 -> Switch16/1
  [VTQD_SpdCtrlLongP_flg] -> Speed Control Mode/3(VTQD_SpdCtrlLongP_flg)
  Switch13/1 -> Switch15/1
  Switch16/1 -> [VTQD_SWCCancelSta_flg], VTQD_SWCCancelSta_flg/1  "VTQD_SWCCancelSta_flg"
  [VTQD_SpdCtrlShortP_flg] -> Speed Control Mode/2(VTQD_SpdCtrlShortP_flg)
  [VTQD_SWCSetdownSta_flg] -> Speed Setting Mode/9(VTQD_SWCSetDownSta_flg)
  [VTQD_SWCACCSta_flg] -> SpdCtrlBotton Behavior/1(SWC_ACC_Sta)
  SpdCtrlBotton Behavior/1(VTQD_SpdCtrlShortP_flg) -> [VTQD_SpdCtrlShortP_flg]  "VTQD_SpdCtrlShortP_flg"
  VDDM_SWCCANCELSta_flg/1 -> Switch16/2
  Constant78/1 -> Switch13/1
  Constant94/1 -> Switch26/1
  VVMC_LVDAACCStatusInformation_flg/1 -> Speed Setting Mode/12(VVMC_LVDAACCStatusInformation_flg)
  [VTQD_SWCCancelSta_flg] -> Speed Setting Mode/10(VTQD_SWCCancelSta_flg)
  VINP_SWCCANCELSta_flg/1 -> Switch16/3
  VTQD_IVIISAOffsetSpdCHOOSE_flg/1(VTQD_IVIISAOffsetSpdCHOOSE_flg) -> [VTQD_IVIISAOffsetSpdCHOOSE_flg]
  Speed Control Mode/1(VTQD_SpdCtrlMode_enum) -> Switch13/3
  [VPMM_PowerSta_enum] -> Equal30/1
  VVMC_MeterIndSpeed_raw32/1 -> Speed Setting Mode/14(VVMC_MeterIndSpeed_raw32)
  Switch23/1 -> [VTQD_SWCResUpSta_flg], VTQD_SWCResUpSta_flg/1  "VTQD_SWCResUpSta_flg"
  Switch25/1 -> [VTQD_SWCSetdownSta_flg], VTQD_SWCSetdownSta_flg/1  "VTQD_SWCSetdownSta_flg"
  VVMC_SetACCDisableAPS_flg/1 -> Speed Setting Mode/17(VVMC_SetACCDisableAPS_flg)
  [VTQD_IVIISAOffsetSpdCHOOSE_flg] -> Speed Control Mode/6(VTQD_IVIISAOffsetSpdCHOOSE_flg)
  Equal30/1 -> Switch15/2
  VINP_Distanceunit_flg/1 -> Speed Setting Mode/15(VINP_Distanceunit_flg)
  Constant90/1 -> Equal30/2
  VTQD_IVIISAOffsetSpd_enum/1 -> VTQD_IVIISAOffsetSpdCHOOSE_flg/1(VTQD_IVIISAOffsetSpd_enum)
  VINP_SWCSetdownSta_flg/1 -> Switch25/3
  VDDM_SWCSetdownSta_flg/1 -> Switch25/2
  VINP_SmartEcoModeSW_flg/1 -> Speed Setting Mode/16(VINP_SmartEcoModeSW_flg)
  Speed Control Mode/2(VTQD_SpdCtrlSta_flg) -> VTQD_SWCSpdCtrlSta_flg/1  "VTQD_SWCSpdCtrlSta_flg"
  Switch15/1 -> [VTQD_SpdCtrlMode_enum], VTQD_SWCSpdCtrlMode_enum/1  "VTQD_SWCSpdCtrlMode_enum"
  VVMC_MSACtrlSta_enum/1 -> Speed Setting Mode/6(VVMC_MSACtrlSta_enum)
  VVMC_CCCtrlSta_enum/1 -> Speed Setting Mode/5(VVMC_CCCtrlSta_enum)
  Data Type Conversion4/1 -> VTQD_SWCSetSpd_kph/1
  task_time_s/1 -> [task_time_s]
  [task_time_s] -> Speed Setting Mode/11(task_time_s)
  VTQD_ShiftGearPosn_enum/1 -> [VTQD_ShiftGearPosn_enum]
  [VTQD_ShiftGearPosn_enum] -> Speed Control Mode/7(VTQD_ShiftGearPosn_enum)
  [VTQD_ShiftGearPosn_enum] -> Speed Setting Mode/2(VTQD_ShiftGearPosn_enum)
  VPMM_PowerSta_enum/1 -> [VPMM_PowerSta_enum]
  [VPMM_PowerSta_enum] -> Speed Control Mode/1(VPMM_PowerSta_enum)
  [VPMM_PowerSta_enum] -> Speed Setting Mode/1(VPMM_PowerSta_enum)
  VINP_ADASACCSta_enum/1 -> [VINP_ADASACCSta_enum]
  [VINP_ADASACCSta_enum] -> Speed Control Mode/4(VINP_ADASACCSta_enum)
  [VINP_ADASACCSta_enum] -> Speed Setting Mode/4(VINP_ADASACCSta_enum)
  Switch24/1 -> Terminator/1  "VTQD_CalMeterSpeed_kph"
  Vehicle to Meter Speed/1(OutputSpeed) -> Switch24/1
  Relational Operator6/1 -> AND6/2
  Relational Operator2/1 -> AND6/1
  [VINP_VehSpeed_kph] -> Vehicle to Meter Speed/1(InputSpeed)
  Constant82/1 -> Relational Operator2/2
  [VINP_VehSpeed_kph] -> Switch24/3
  [VINP_VehSpeed_kph] -> Relational Operator2/1
  [VINP_VehSpeed_kph] -> Relational Operator6/1
  AND6/1 -> Switch24/2
  Constant84/1 -> Relational Operator6/2
  VINP_VehSpeed_kph/1 -> [VINP_VehSpeed_kph]
  Speed Setting Mode/2(VTQD_SetSpdLimWarn_flg) -> VTQD_SWCSetSpdLimWarn_flg/1
  Speed Setting Mode/6(VTQD_SWCISASetSpd_kph) -> VTQD_SWCISASetSpd_kph/1
  Speed Setting Mode/3(VTQD_SWCACCSetSpd_kph) -> VTQD_SWCACCSetSpd_kph/1
  Speed Setting Mode/4(VTQD_SWCCCSetSpd_kph) -> VTQD_SWCCCSetSpd_kph/1
  Speed Setting Mode/5(VTQD_SWCMSASetSpd_kph) -> VTQD_SWCMSASetSpd_kph/1
  Speed Setting Mode/7(VTQD_SWCAllowSetSpd_flg) -> VTQD_SWCAllowSetSpd_flg/1
  Speed Setting Mode/8(VTQD_SWCCCSpdResetFinish_flg) -> VTQD_SWCCCSpdResetFinish_flg/1

== system tqd/TQD/TorqueDemand/Signal_convert/Simulation Sound Wave  ==
  note: Simulation Sound Wave Request
  note: Simulation Sound Wave Command
  note: System Performance
  note: System Torque Power
  note: System Motor Power
  VTQD_ActAPSPosn_pct : Inport
  VINP_FrTMSpd_rpm : Inport  Port=2
  VINP_RrTMSpd_rpm : Inport  Port=3
  VINP_FrEDURealTMTq_Nm : Inport  Port=4
  VINP_RrEDURealTMTq_Nm : Inport  Port=5
  VTQD_GearActualPosn_enum : Inport  Port=6
  task_time_s : Inport  Port=7
  Abs : Abs
  Abs1 : Abs
  Add{,1..4} (5 alike) : Sum
  Constant : Constant  Value=PI
  Constant1 : Constant  Value=TWO_FLOAT
  Constant{3,5,10,15} (4 alike) : Constant  Value=EPS
  Constant11 : Constant  Value=KTQD_FrMotorRefPower_kW
  Constant12 : Constant  Value=ENUM_GEARACTUALPOSN_R
  Constant13 : Constant  Value=KTQD_FrUppTheldTrq_Nm
  Constant14 : Constant  Value=KTQD_RrUppTheldTrq_Nm
  Constant16 : Constant  Value=KTQD_SimSoundWaveSet_enum
  Constant17 : Constant  Value=ONE_INT
  Constant18 : Constant  Value=KTQD_SimSoundWaveSet_enum
  Constant19 : Constant  Value=TWO_INT
  Constant2 : Constant  Value=SIXTY
  Constant20 : Constant  Value=KTQD_SimSoundWaveSet_enum
  Constant21 : Constant  Value=THREE_INT
  Constant22 : Constant  Value=ZERO_FLOAT
  Constant23 : Constant  Value=KTQD_SimSoundWaveInc_pct
  Constant24 : Constant  Value=KTQD_SimSoundWaveDec_pct
  Constant4 : Constant  Value=KTQD_RrMotorRefPower_kW
  Constant6 : Constant  Value=THOUSAND
  Constant7 : Constant  Value=PI
  Constant8 : Constant  Value=TWO_FLOAT
  Constant9 : Constant  Value=SIXTY
  Divide{,1..3} (4 alike) : Product  Inputs=*/
  Equal{,1..3} (4 alike) : RelationalOperator  Operator===  OutDataTypeStr=boolean  RndMeth=Simplest
  Gain : Gain  Gain=HUNDRED
  Gain2 : Gain  Gain=HUNDRED
  MINUSONE_FLOAT : Gain  Gain=MINUSONE_FLOAT
  Max{,1..3} (4 alike) : MinMax  Function=max  Inputs=2
  Product : Product  Inputs=4
  Product1 : Product
  Product2 : Product  Inputs=4
  RateLimit : hcu_lib/Basic_Blocks/RateLimit
  Relational Operator : RelationalOperator  OutDataTypeStr=boolean  RndMeth=Simplest
  Switch{,1..4} (5 alike) : Switch  Criteria=u2 ~= 0
      settings: AttributesFormatString=%<Criteria>
  VTQD_SimSouWaveReq_pct : Outport
  wires:
  Constant/1 -> Product/3
  Add1/1 -> Divide2/1
  Constant19/1 -> Equal2/2
  Constant2/1 -> Max/1
  Constant23/1 -> RateLimit/4
  Max3/1 -> Divide3/2
  Product1/1 -> Max1/1
  [VINP_RrTMSpd_rpm] -> Product2/2
  Divide/1 -> [VTQD_FrMotorPwr_W]  "VTQD_FrMotorPwr_W"
  Constant18/1 -> Equal2/1
  Constant7/1 -> Product2/3
  VTQD_ActAPSPosn_pct/1 -> [VTQD_ActAPSPosn_pct]
  MINUSONE_FLOAT/1 -> Switch/1
  Switch1/1 -> Switch2/3
  [VINP_FrEDURealTMTq_Nm] -> Add3/1
  [VINP_RrEDURealTMTq_Nm] -> Add2/2
  Constant12/1 -> Equal/2
  Divide2/1 -> Gain/1
  VINP_RrEDURealTMTq_Nm/1 -> [VINP_RrEDURealTMTq_Nm]
  [VINP_FrEDURealTMTq_Nm] -> Product/1
  Switch3/1 -> [VTQD_SimSouWaveCMD_pct]  "VTQD_SimSouWaveCMD_pct"
  Constant20/1 -> Equal3/1
  Constant17/1 -> Equal1/2
  Constant22/1 -> RateLimit/2
  [VTQD_SysMotorPerform_pct] -> Switch3/1
  [VTQD_SysMotorTorque_pct] -> Abs1/1
  Equal2/1 -> Switch2/2
  Abs1/1 -> Relational Operator/2
  [VTQD_FrMotorPwr_W] -> Add1/1
  Add/1 -> Product1/1
  Gain2/1 -> [VTQD_SysMotorTorque_pct]  "VTQD_SysMotorTorque_pct"
  Constant4/1 -> Add/2
  [VTQD_SysMotorPower_pct] -> Switch4/1
  Constant11/1 -> Add/1
  Divide3/1 -> Gain2/1
  Switch4/1 -> [VTQD_SysMotorPerform_pct]  "VTQD_SysMotorPerform_pct"
  [VTQD_SimSouWaveCMD_pct] -> RateLimit/1
  Equal/1 -> Switch/2
  [VTQD_SysMotorPower_pct] -> Switch2/1
  task_time_s/1 -> [task_time_s]
  VINP_RrTMSpd_rpm/1 -> [VINP_RrTMSpd_rpm]
  Add4/1 -> Max3/1
  Switch2/1 -> Switch3/3
  Gain/1 -> [VTQD_SysMotorPower_pct]  "VTQD_SysMotorPower_pct"
  Constant16/1 -> Equal1/1
  Constant24/1 -> RateLimit/5
  [VTQD_ActAPSPosn_pct] -> Switch1/3
  [VINP_FrEDURealTMTq_Nm] -> Add2/1
  Constant6/1 -> Product1/2
  Constant1/1 -> Product/4
  [VINP_RrEDURealTMTq_Nm] -> Add3/2
  Equal3/1 -> Switch3/2
  [VTQD_SysMotorPower_pct] -> Abs/1
  Constant13/1 -> Add4/1
  [VINP_FrTMSpd_rpm] -> Product/2
  Constant5/1 -> Max1/2
  Constant3/1 -> Max/2
  [VTQD_SysMotorTorque_pct] -> Switch1/1
  Constant15/1 -> Max3/2
  Constant21/1 -> Equal3/2
  Product/1 -> Divide/1
  VINP_FrTMSpd_rpm/1 -> [VINP_FrTMSpd_rpm]
  Add3/1 -> Switch/3
  [VTQD_RrMotorPwr_W] -> Add1/2
  Relational Operator/1 -> Switch4/2
  Add2/1 -> MINUSONE_FLOAT/1
  Abs/1 -> Relational Operator/1
  RateLimit/1 -> [VTQD_SimSouWaveReq_pct]  "VTQD_SimSouWaveReq_pct"
  Max1/1 -> Divide2/2
  Equal1/1 -> Switch1/2
  VINP_FrEDURealTMTq_Nm/1 -> [VINP_FrEDURealTMTq_Nm]
  [VTQD_SimSouWaveReq_pct] -> VTQD_SimSouWaveReq_pct/1
  [VTQD_SysMotorTorque_pct] -> Switch4/3
  [task_time_s] -> RateLimit/3
  Switch/1 -> Divide3/1
  [VTQD_GearActualPosn_enum] -> Equal/1
  Constant14/1 -> Add4/2
  Max/1 -> Divide/2
  [VINP_RrEDURealTMTq_Nm] -> Product2/1
  Constant8/1 -> Product2/4
  Divide1/1 -> [VTQD_RrMotorPwr_W]  "VTQD_RrMotorPwr_W"
  Constant10/1 -> Max2/2
  Max2/1 -> Divide1/2
  Constant9/1 -> Max2/1
  Product2/1 -> Divide1/1
  VTQD_GearActualPosn_enum/1 -> [VTQD_GearActualPosn_enum]

== system tqd/TQD/TorqueDemand/Signal_convert/Subsystem ==
  note: Shifter1 message
  note: CNA3
  VINP_ShifterHandleCmd_enum : Inport
  VINP_ShifterFailsta_enum : Inport  Port=2
  VDDM_Shifter1Err_flg : Inport  Port=3
  Constant24 : Constant  Value=KTQD_VirtualShifterCMD_enum
  Constant25 : Constant  Value=KTQD_ShifterInvalidSW_flg  OutDataTypeStr=single
  Constant26 : Constant  Value=0xFF  OutDataTypeStr=single
  Constant27 : Constant  Value=ENUM_SHIFTERERRSTA_SHIFTERFAILURE
  Constant28 : Constant  Value=KTQD_ShifterInvalidSW_flg  OutDataTypeStr=single
  Equal8 : RelationalOperator  OutDataTypeStr=boolean  RndMeth=Simplest
  Logical Operator16 : Logic  Operator=OR  AllPortsSameDT=off  OutDataTypeStr=boolean
  Logical Operator17 : Logic  AllPortsSameDT=off  OutDataTypeStr=boolean
  Logical Operator19 : Logic  AllPortsSameDT=off  OutDataTypeStr=boolean
  Switch8 : Switch  Criteria=u2 ~= 0
  Switch9 : Switch  Criteria=u2 ~= 0
  VTQD_ShifterHandleCmd_enum : Outport
  VTQD_ShifterFailsta_enum : Outport  Port=2
  wires:
  Constant25/1 -> Logical Operator17/2
  Constant28/1 -> Logical Operator19/2
  Constant26/1 -> Equal8/2
  Constant27/1 -> Switch9/1
  Switch9/1 -> [VTQD_ShifterFailsta_enum]  "VTQD_ShifterFailsta_enum"
  Constant24/1 -> Switch8/1
  [VINP_ShifterFailsta_enum] -> Switch9/3
  Logical Operator19/1 -> Switch9/2
  [VDDM_Shifter1Err_flg] -> Logical Operator19/1
  Logical Operator16/1 -> Logical Operator17/1
  Equal8/1 -> Logical Operator16/2
  [VINP_ShifterHandleCmd_enum] -> Equal8/1
  [VINP_ShifterHandleCmd_enum] -> Switch8/3
  Switch8/1 -> [VTQD_ShifterHandleCmd_enum]  "VTQD_ShifterHandleCmd_enum"
  Logical Operator17/1 -> Switch8/2
  VINP_ShifterHandleCmd_enum/1 -> [VINP_ShifterHandleCmd_enum]
  VINP_ShifterFailsta_enum/1 -> [VINP_ShifterFailsta_enum]
  [VTQD_ShifterHandleCmd_enum] -> VTQD_ShifterHandleCmd_enum/1
  [VTQD_ShifterFailsta_enum] -> VTQD_ShifterFailsta_enum/1
  VDDM_Shifter1Err_flg/1 -> [VDDM_Shifter1Err_flg]
  [VDDM_Shifter1Err_flg] -> Logical Operator16/1

== system tqd/TQD/TorqueDemand/Signal_convert/VehWeightEst ==
  VTQD_AfterAvailableTqDemRr_Nm : Inport
  VTQR_NoABSREDUWhlTqReq_Nm : Inport  Port=2
  VTQR_NoABSFEDUWhlTqReq_Nm : Inport  Port=3
  VTQD_AfterAvailableTqDemFr_Nm : Inport  Port=4
  VTQD_GearActualPosn_enum : Inport  Port=5
  VINP_VehSpeed_kph : Inport  Port=6
  VTQD_RollRegenDisableReq_flg : Inport  Port=7
  VINP_RegenMode_enum : Inport  Port=8
  VTQD_LowIdleAccPedal_flg : Inport  Port=9
  VTQD_BrkSwSta_flg : Inport  Port=10
  VINP_RrRBCActive_flg : Inport  Port=11
  VINP_FrRBCActive_flg : Inport  Port=12
  VINP_GRADE_Deg : Inport  Port=13
  task_time_s : Inport  Port=14
  VVMC_LongAcc_Gps : Inport  Port=15
  VINP_FrEDURealTMTq_Nm : Inport  Port=16
  VINP_RrEDURealTMTq_Nm : Inport  Port=17
  VINP_DriverSeatBeltCmd_flg : Inport  Port=18
  VINP_PsngrSeatBeltCmd_flg : Inport  Port=19
  VINP_RDriverSeatBeltCmd_flg : Inport  Port=20
  VINP_RCenterSeatBeltCmd_flg : Inport  Port=21
  VINP_RPsngrSeatBeltCmd_flg : Inport  Port=22
  Calaulation : Subsystem
  Condition : Subsystem
  Desicion : Subsystem
  VTQD_EstVehWeightResult_kg : Outport
  wires:
  Calaulation/2(VTQD_EstFrRealTqCheckPass_flg) -> [VTQD_EstFrRealTqCheckPass_flg]
  [VTQD_BrkSwSta_flg] -> Condition/10(VTQD_BrkSwSta_flg)
  Condition/2(VTQD_VehWeightEstDis_flg) -> [VTQD_VehWeightEstDis_flg]
  VTQD_RollRegenDisableReq_flg/1 -> [VTQD_RollRegenDisableReq_flg]
  [VINP_VehSpeed_kph] -> Calaulation/8(VINP_VehSpeed_kph)
  [VINP_PsngrSeatBeltCmd_flg] -> Desicion/5(VINP_PsngrSeatBeltCmd_flg)
  VTQD_BrkSwSta_flg/1 -> [VTQD_BrkSwSta_flg]
  [task_time_s] -> Calaulation/1(task_time_s)
  [VINP_RCenterSeatBeltCmd_flg] -> Desicion/7(VINP_RCenterSeatBeltCmd_flg)
  [VINP_FrEDURealTMTq_Nm] -> Calaulation/6(VINP_FrEDURealTMTq_Nm)
  VINP_RrEDURealTMTq_Nm/1 -> [VINP_RrEDURealTMTq_Nm]
  [VTQD_VehWeightEstEnd_flg] -> Calaulation/4(VTQD_VehWeightEstEnd_flg)
  [VTQR_NoABSREDUWhlTqReq_Nm] -> Condition/2(VTQR_NoABSREDUWhlTqReq_Nm)
  [VTQD_VehWeightEstDis_flg] -> Calaulation/3(VTQD_VehWeightEstDis_flg)
  [VVMC_LongAcc_Gps] -> Calaulation/5(VVMC_LongAcc_Gps)
  VTQD_GearActualPosn_enum/1 -> [VTQD_GearActualPosn_enum]
  [VTQD_EstRrRealTqCheckPass_flg] -> Desicion/11(VTQD_EstRrRealTqCheckPass_flg)
  VINP_RCenterSeatBeltCmd_flg/1 -> [VINP_RCenterSeatBeltCmd_flg]
  [VTQD_EstVehWeightResult_kg] -> VTQD_EstVehWeightResult_kg/1
  [VTQD_RollRegenDisableReq_flg] -> Condition/7(VTQD_RollRegenDisableReq_flg)
  [VINP_RPsngrSeatBeltCmd_flg] -> Desicion/8(VINP_RPsngrSeatBeltCmd_flg)
  [VTQD_VehWeightEstEn_flg] -> Calaulation/2(VTQD_VehWeightEstEn_flg)
  VINP_GRADE_Deg/1 -> [VINP_GRADE_Deg]
  VTQD_AfterAvailableTqDemRr_Nm/1 -> [VTQD_AfterAvailableTqDemRr_Nm]
  [VINP_RegenMode_enum] -> Condition/8(VINP_RegenMode_enum)
  task_time_s/1 -> [task_time_s]
  [VTQD_EstLongAccCheckPass_flg] -> Desicion/9(VTQD_EstLongAccCheckPass_flg)
  [VTQD_LowIdleAccPedal_flg] -> Condition/9(VTQD_LowIdleAccPedal_flg)
  VINP_RPsngrSeatBeltCmd_flg/1 -> [VINP_RPsngrSeatBeltCmd_flg]
  [VTQD_GearActualPosn_enum] -> Condition/5(VTQD_GearActualPosn_enum)
  [VINP_RrRBCActive_flg] -> Condition/11(VINP_RrRBCActive_flg)
  Condition/1(VTQD_VehWeightEstEn_flg) -> [VTQD_VehWeightEstEn_flg]
  Desicion/1(VTQD_VehWeightEstEnd_flg) -> [VTQD_VehWeightEstEnd_flg]
  [VINP_DriverSeatBeltCmd_flg] -> Desicion/4(VINP_DriverSeatBeltCmd_flg)
  [VTQD_VehWeightEstDis_flg] -> Desicion/2(VTQD_VehWeightEstDis_flg)
  VINP_DriverSeatBeltCmd_flg/1 -> [VINP_DriverSeatBeltCmd_flg]
  VINP_VehSpeed_kph/1 -> [VINP_VehSpeed_kph]
  [task_time_s] -> Condition/14(task_time_s)
  VTQR_NoABSREDUWhlTqReq_Nm/1 -> [VTQR_NoABSREDUWhlTqReq_Nm]
  [VINP_RrEDURealTMTq_Nm] -> Calaulation/7(VINP_RrEDURealTMTq_Nm)
  [VTQR_NoABSFEDUWhlTqReq_Nm] -> Condition/3(VTQR_NoABSFEDUWhlTqReq_Nm)
  [VTQD_AfterAvailableTqDemFr_Nm] -> Condition/4(VTQD_AfterAvailableTqDemFr_Nm)
  VINP_RrRBCActive_flg/1 -> [VINP_RrRBCActive_flg]
  [VINP_FrRBCActive_flg] -> Condition/12(VINP_FrRBCActive_flg)
  VTQD_AfterAvailableTqDemFr_Nm/1 -> [VTQD_AfterAvailableTqDemFr_Nm]
  VINP_FrEDURealTMTq_Nm/1 -> [VINP_FrEDURealTMTq_Nm]
  VTQD_LowIdleAccPedal_flg/1 -> [VTQD_LowIdleAccPedal_flg]
  [VTQD_AfterAvailableTqDemRr_Nm] -> Condition/1(VTQD_AfterAvailableTqDemRr_Nm)
  [VINP_GRADE_Deg] -> Condition/13(VINP_GRADE_Deg)
  [VINP_VehSpeed_kph] -> Condition/6(VINP_VehSpeed_kph)
  VINP_RegenMode_enum/1 -> [VINP_RegenMode_enum]
  VTQR_NoABSFEDUWhlTqReq_Nm/1 -> [VTQR_NoABSFEDUWhlTqReq_Nm]
  VINP_RDriverSeatBeltCmd_flg/1 -> [VINP_RDriverSeatBeltCmd_flg]
  VINP_PsngrSeatBeltCmd_flg/1 -> [VINP_PsngrSeatBeltCmd_flg]
  Calaulation/3(VTQD_EstRrRealTqCheckPass_flg) -> [VTQD_EstRrRealTqCheckPass_flg]
  [VTQD_EstFrRealTqCheckPass_flg] -> Desicion/10(VTQD_EstFrRealTqCheckPass_flg)
  Calaulation/1(VTQD_EstLongAccCheckPass_flg) -> [VTQD_EstLongAccCheckPass_flg]
  VVMC_LongAcc_Gps/1 -> [VVMC_LongAcc_Gps]
  [VTQD_VehWeightEstEnd_flg] -> Condition/15(VTQD_VehWeightEstEnd_flg)
  [VINP_RDriverSeatBeltCmd_flg] -> Desicion/6(VINP_RDriverSeatBeltCmd_flg)
  [VTQD_EstVehWeight_kg] -> Desicion/3(VTQD_EstVehWeight_kg)
  Calaulation/4(VTQD_EstVehWeight_kg) -> [VTQD_EstVehWeight_kg]
  Desicion/2(VTQD_EstVehWeightResult_kg) -> [VTQD_EstVehWeightResult_kg]
  [task_time_s] -> Desicion/1(task_time_s)
  VINP_FrRBCActive_flg/1 -> [VINP_FrRBCActive_flg]
